simulink model "Controllo2_1"  (Simulink 7.8)
settings: Solver=ode23s  StartTime=0.0  StopTime=250  RelTol=1e-10
values from neighbouring files (symbols this model uses):
  f = 0.9*10^5    (= 90000)    [Controllo_rollio_natante.m]
  h = m*g*(b-a)    (= 725940)    [Controllo_rollio_natante.m]
  J = 0.16*10^7    (= 1600000)    [Controllo_rollio_natante.m]
  Km = 1    [Controllo_rollio_natante.m]
  La = 0.025    [Controllo_rollio_natante.m]
  Ra = 0.30    (= 0.3)    [Controllo_rollio_natante.m]
settings Model: Creator=dAnIeLe  LastModifiedBy=dAnIeLe

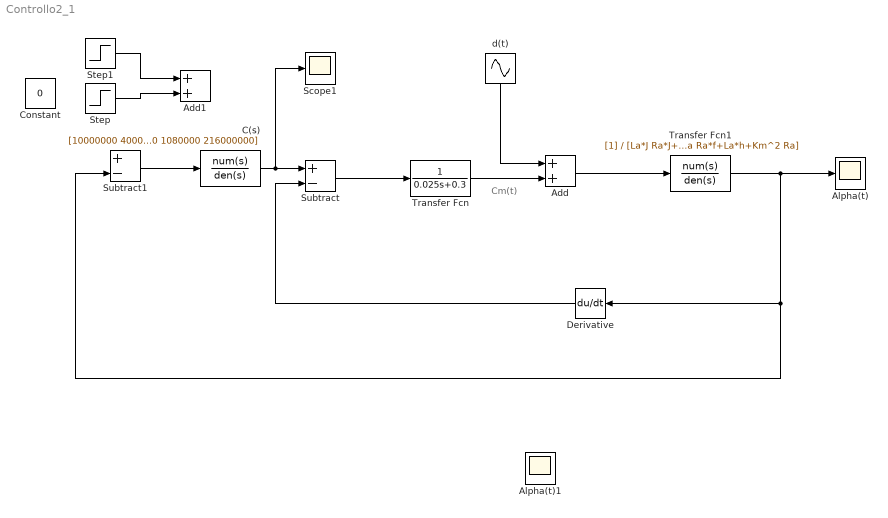
== system Controllo2_1 ==
  note: Cm(t)
  Add : Sum
  Add1 : Sum
  Alpha(t) : Scope
      settings: TimeRange=7  YMin=0.003  YMax=0.00405
  Alpha(t)1 : Scope
      settings: TimeRange=7  YMin=0.003  YMax=0.00405  SaveName=ScopeData2
  C(s) : TransferFcn  Numerator=[10000000 4000000 4000000]  Denominator=[1 1800 1080000 216000000]
  Constant : Constant  Value=0
  Derivative : Derivative
  Scope1 : Scope
  Step : Step  Time=0  SampleTime=0
  Step1 : Step  Time=0.5  Before=1  After=0  SampleTime=0
  Subtract : Sum  Inputs=+-
  Subtract1 : Sum  Inputs=+-
  Transfer Fcn : TransferFcn  Denominator=[0.025 0.3]
  Transfer Fcn1 : TransferFcn  Denominator=[La*J Ra*J+f*La Ra*f+La*h+Km^2 Ra]
  d(t) : Sin  Amplitude=100  Frequency=0.628  SampleTime=0
  wires:
  Subtract1/1 -> C(s)/1
  C(s)/1 -> Subtract/1, Scope1/1
  Subtract/1 -> Transfer Fcn/1
  Transfer Fcn/1 -> Add/2
  Add/1 -> Transfer Fcn1/1
  Transfer Fcn1/1 -> Alpha(t)/1, Derivative/1, Subtract1/2
  Derivative/1 -> Subtract/2
  Step1/1 -> Add1/1
  Step/1 -> Add1/2
  d(t)/1 -> Add/1
